simulink model "uwb_6_delay_mult_optim"  (R2025a)
settings: Solver=VariableStepAuto  StartTime=0.0  StopTime=1.5e-6  RelTol=1e-3
undefined symbols (not defined in the file or in its folder): j
libraries: simulink_extras x2, commrfcorlib x1, commchan3 x1, commdigbbndpm3 x1, dspstat3 x1
settings Model: Creator=IWMAI  LastModifiedBy=IWMAI

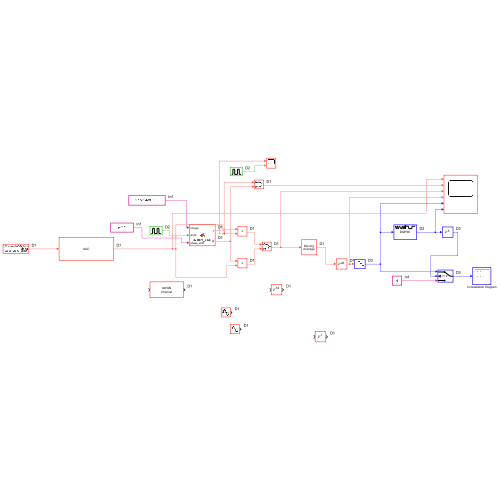
[thumbnail: Simulink's stored preview of the top-level diagram]
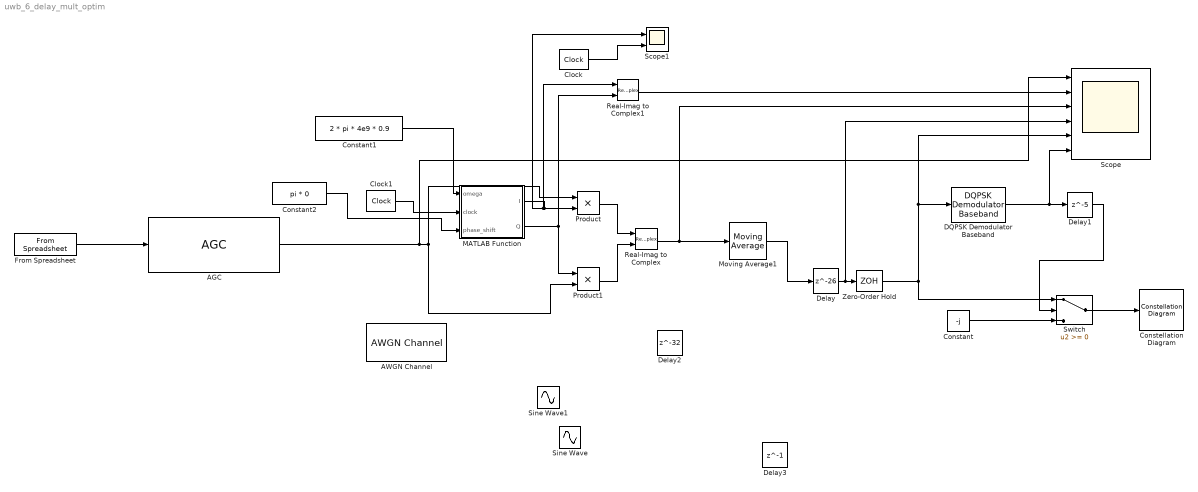
== system uwb_6_delay_mult_optim ==
  AGC : commrfcorlib/AGC  LegacyMode=off  DetectorMethod=Rectifier  LoopMethod=Linear  UpdatePeriod=100  StepSize=0.1  AdaptationStepSize=0.01  DesiredOutputPower=1  AveragingLength=64  MaximumGain=30  MaxPowerGain=60  GainOutputPort=off  InputPowerOutputPort=off  SimulateUsing=Interpreted execution
  AWGN Channel : commchan3/AWGN Channel  LegacyMode=off  NoiseMethod="Signal to noise ratio  (SNR)"  noiseMode="Signal to noise ratio  (SNR)"  EbNo=10  EsNo=10  SNR=10  BitsPerSymbol=1  SignalPower=1  SpecifySymbolPeriod=off  SamplesPerSymbol=1  SymbolPeriod=1  VarianceSource=Parameter  Variance=1  RandomStream=mt19937ar with seed  Seed=67  SimulateUsing=Code generation
  Clock : simulink_extras/Flip Flops/Clock  period=1/500e6
  Clock1 : simulink_extras/Flip Flops/Clock  period=1/500e6
  Constant : Constant  Value=-j
  Constant1 : Constant  Value=2 * pi * 4e9 * 0.9
  Constant2 : Constant  Value=pi * 0
  Constellation Diagram : ConstellationDiagram  WindowPosition=[-1706.000000,-29.000000,1707.000000,996.000000,]  Visible=on  ScopeFrameLocation=window  SymbolsToDisplaySource=Property  SymbolsToDisplay=2500  ReferenceConstellation=QPSK  XLimits=[-2.067197093509777,2.1540515483355467]  YLimits=[-2.067197093509777,2.1540515483355467]  AxesLimits=[-2.067197093509777,2.1540515483355467]  EnableMeasurements=on  DefaultConfigurationName=comm.scopes.ConstellationDiagramBlockCfg
  DQPSK Demodulator Baseband : commdigbbndpm3/DQPSK Demodulator Baseband  OutType=Integer  Dec=Gray  Ph=0  outDtype1=Inherit via internal rule  outDtype2=Inherit via internal rule
  Delay : Delay  DelayLength=26
  Delay1 : Delay  DelayLength=5  InitialCondition=-1
  Delay2 : Delay  DelayLength=32
  Delay3 : Delay  DelayLength=1
  From Spreadsheet : FromSpreadsheet  FileName=C:\Users\IWMAI\University of Toronto\Yu Huang - Summer-2025-sharted\Yongkang\v3_250617\csv\data_zero_time.csv  SheetName=data_zero_time  SampleTime=1/16e9  ExtrapolationBeforeFirstDataPoint=Hold first value  InterpolationWithinTimeRange=Zero order hold  ExtrapolationAfterLastDataPoint=Hold last value
  MATLAB Function : MATLAB Function  TreatAsAtomicUnit=on  SystemSampleTime=1/16e9
  Moving Average1 : dspstat3/Moving Average  Method=Sliding window  ForgettingFactorPort=off  SpecifyWindowLength=on  WindowLength=8  OverlapLength=7  AllowArbitraryInputLength=off  ForgettingFactor=0.9  SimulateUsing=Interpreted execution
  Product : Product
  Product1 : Product
  Real-Imag to Complex : RealImagToComplex
  Real-Imag to Complex1 : RealImagToComplex
  Scope : Scope  NumInputPorts=6
      settings: ActiveDisplayYMinimum=-2.8853361781018032  ActiveDisplayYMaximum=2.6693087362148233
  Scope1 : Scope  NumInputPorts=2
      settings: ActiveDisplayYMinimum=-1.2499999999999791  ActiveDisplayYMaximum=1.2499999999999976
  Sine Wave : Sin  Frequency=2 * pi * 4e9 * 1.005  SampleTime=1/16e9
  Sine Wave1 : Sin  Frequency=2 * pi * 4e9  Phase=pi / 2  SampleTime=1/16e9
  Switch : Switch  SaturateOnIntegerOverflow=off  InputSameDT=off
  Zero-Order Hold : ZeroOrderHold  SampleTime=1/500e6
  wires:
  MATLAB Function/1(I) -> Scope1/1, Real-Imag to Complex1/1, Product/2
  MATLAB Function/2(Q) -> Product1/1, Real-Imag to Complex1/2
  Product/1 -> Real-Imag to Complex/1
  Product1/1 -> Real-Imag to Complex/2
  Real-Imag to Complex/1 -> Scope/3, Moving Average1/1
  Moving Average1/1 -> Delay/1
  Zero-Order Hold/1 -> Switch/1, DQPSK Demodulator Baseband/1, Scope/5
  Delay/1 -> Scope/4, Zero-Order Hold/1
  DQPSK Demodulator Baseband/1 -> Delay1/1, Scope/6
  Real-Imag to Complex1/1 -> Scope/2
  From Spreadsheet/1 -> AGC/1
  AGC/1 -> Scope/1, Product/1, Product1/2
  Delay1/1 -> Switch/2
  Switch/1 -> Constellation Diagram/1
  Constant/1 -> Switch/3
  Clock/1 -> Scope1/2
  Constant1/1 -> MATLAB Function/1(omega)
  Clock1/1 -> MATLAB Function/2(clock)
  Constant2/1 -> MATLAB Function/3(phase_shift)

== matlab function uwb_6_delay_mult_optim/MATLAB Function ==
  data: omega input; clock input; I output; phase_shift input; Q output
function [I, Q]= custom_sine(omega, clock, phase_shift)

% around 4GHz sine wave, restart 1/500e6 sec
% currently assume the sample rate is 16S/s

persistent count;
persistent last_clock; % for detecting the falling edge, because we want to reset the wave on the falling edge
delta_time = 1 / 16e9;

if isempty(count)
    count = 0;
    last_clock = 1;
end

if clock == 0 && last_clock == 1 % means we are on a falling edge
    count = 0;
end

phase = count * omega * delta_time + phase_shift;
disp(phase);

I = sin(phase);
Q = cos(phase);

count = count + 1;
last_clock = clock;
